simulink model "PerfectModel"  (R2018b)
settings: Solver=VariableStepAuto  StartTime=0.0  StopTime=25  RelTol=1e-3
settings Model: Creator=olavoie  LastModifiedBy=olavoie

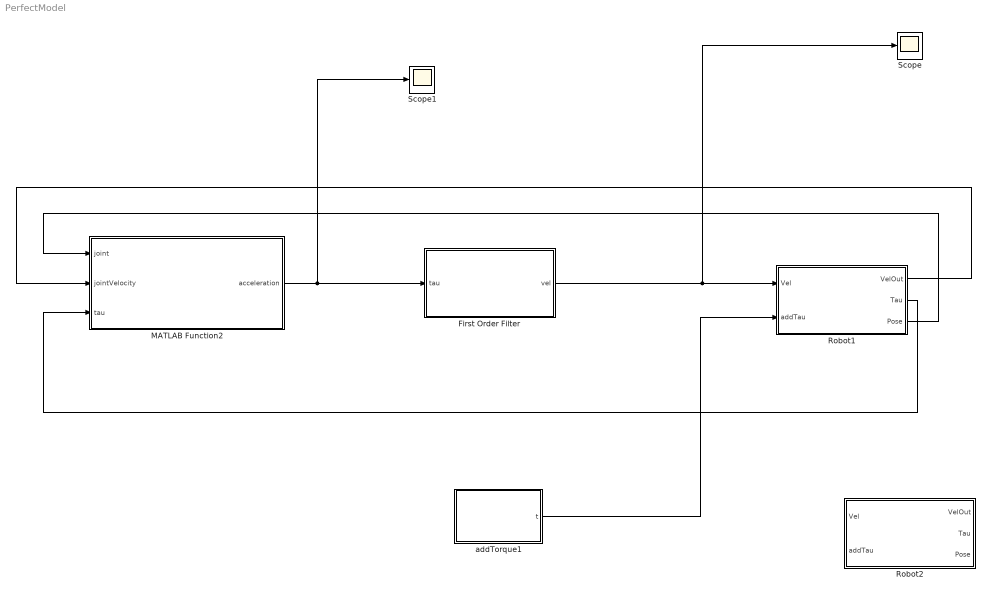
== system PerfectModel ==
  First Order Filter : Subsystem  TreatAsAtomicUnit=on
  MATLAB Function2 : MATLAB Function  TreatAsAtomicUnit=on
  Robot1 : Subsystem  TreatAsAtomicUnit=on
  Robot2 : Subsystem  TreatAsAtomicUnit=on
  Scope : Scope
  Scope1 : Scope
  addTorque1 : Subsystem  TreatAsAtomicUnit=on
  wires:
  MATLAB Function2/1(acceleration) -> Scope1/1, First Order Filter/1(tau)
  First Order Filter/1(vel) -> Scope/1, Robot1/1(Vel)
  Robot1/1(VelOut) -> MATLAB Function2/2(jointVelocity)
  Robot1/3(Pose) -> MATLAB Function2/1(joint)
  Robot1/2(Tau) -> MATLAB Function2/3(tau)
  addTorque1/1(t) -> Robot1/2(addTau)

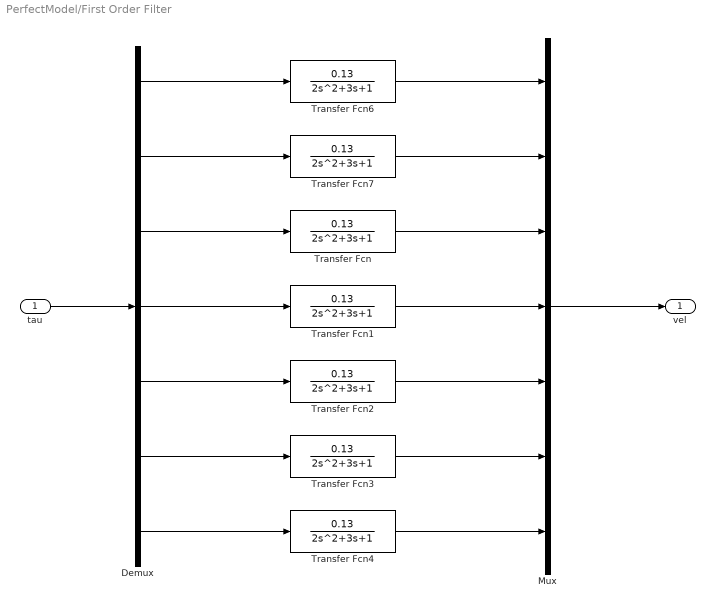
== system PerfectModel/First Order Filter ==
  tau : Inport
  Demux : Demux  Outputs=7
  Mux : Mux  Inputs=7
  Transfer Fcn{,1..4,6..7} (7 alike) : TransferFcn  Numerator=[0.13]  Denominator=[2 3 1]
  vel : Outport
  wires:
  Transfer Fcn2/1 -> Mux/5
  Demux/7 -> Transfer Fcn4/1
  Transfer Fcn1/1 -> Mux/4
  Transfer Fcn4/1 -> Mux/7
  Transfer Fcn/1 -> Mux/3
  Demux/3 -> Transfer Fcn/1
  Demux/5 -> Transfer Fcn2/1
  Transfer Fcn7/1 -> Mux/2
  Transfer Fcn3/1 -> Mux/6
  Mux/1 -> vel/1
  Demux/4 -> Transfer Fcn1/1
  tau/1 -> Demux/1
  Demux/6 -> Transfer Fcn3/1
  Transfer Fcn6/1 -> Mux/1
  Demux/2 -> Transfer Fcn7/1
  Demux/1 -> Transfer Fcn6/1

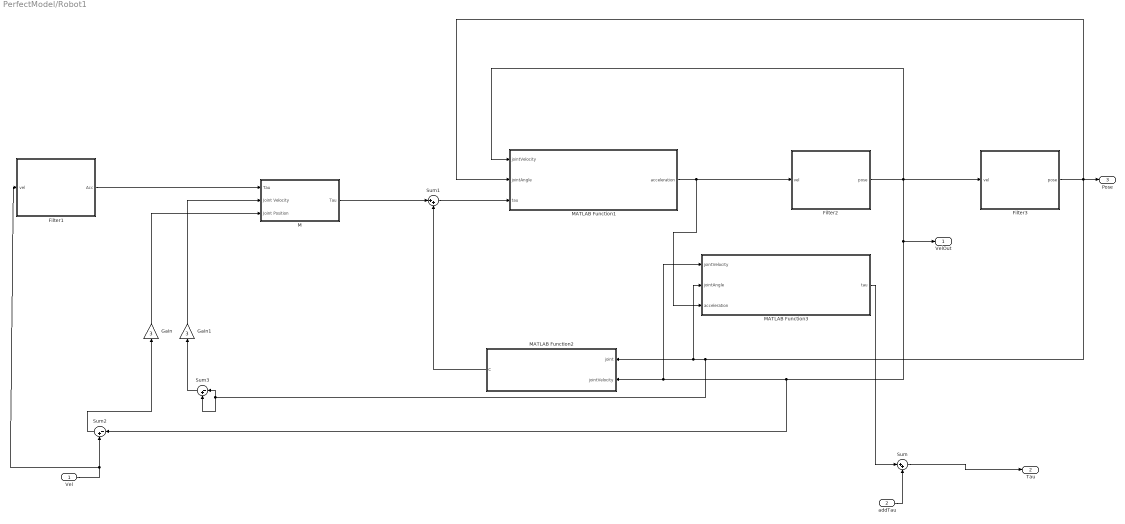
== system PerfectModel/Robot1 ==
  Vel : Inport
  addTau : Inport  Port=2
  Filter1 : Subsystem  TreatAsAtomicUnit=on
  Filter2 : Subsystem  TreatAsAtomicUnit=on
  Filter3 : Subsystem  TreatAsAtomicUnit=on
  Gain : Gain  Gain=3
  Gain1 : Gain  Gain=3
  M : Subsystem  TreatAsAtomicUnit=on
  MATLAB Function1 : MATLAB Function  TreatAsAtomicUnit=on
  MATLAB Function2 : MATLAB Function  TreatAsAtomicUnit=on
  MATLAB Function3 : MATLAB Function  TreatAsAtomicUnit=on
  Sum : Sum  Inputs=|++
  Sum1 : Sum  Inputs=|++
  Sum2 : Sum  Inputs=|-+
  Sum3 : Sum  Inputs=|-+
  VelOut : Outport
  Tau : Outport  Port=2
  Pose : Outport  Port=3
  wires:
  Sum1/1 -> MATLAB Function1/3(tau)
  MATLAB Function1/1(acceleration) -> MATLAB Function3/3(acceleration), Filter2/1(vel)
  Filter2/1(pose) -> VelOut/1, Sum2/1, MATLAB Function3/1(jointVelocity), MATLAB Function2/2(jointVelocity), Filter3/1(vel), MATLAB Function1/1(jointVelocity)
  Filter3/1(pose) -> Sum3/2, Sum3/1, MATLAB Function3/2(jointAngle), MATLAB Function2/1(joint), MATLAB Function1/2(jointAngle), Pose/1
  addTau/1 -> Sum/2
  Sum/1 -> Tau/1
  M/1(Tau) -> Sum1/1
  MATLAB Function2/1(C) -> Sum1/2
  Sum3/1 -> Gain1/1
  Gain1/1 -> M/2(Joint Velocity)
  Sum2/1 -> Gain/1
  Gain/1 -> M/3(Joint Position)
  Vel/1 -> Filter1/1(vel), Sum2/2
  Filter1/1(Acc) -> M/1("Tau ")
  MATLAB Function3/1(tau) -> Sum/1

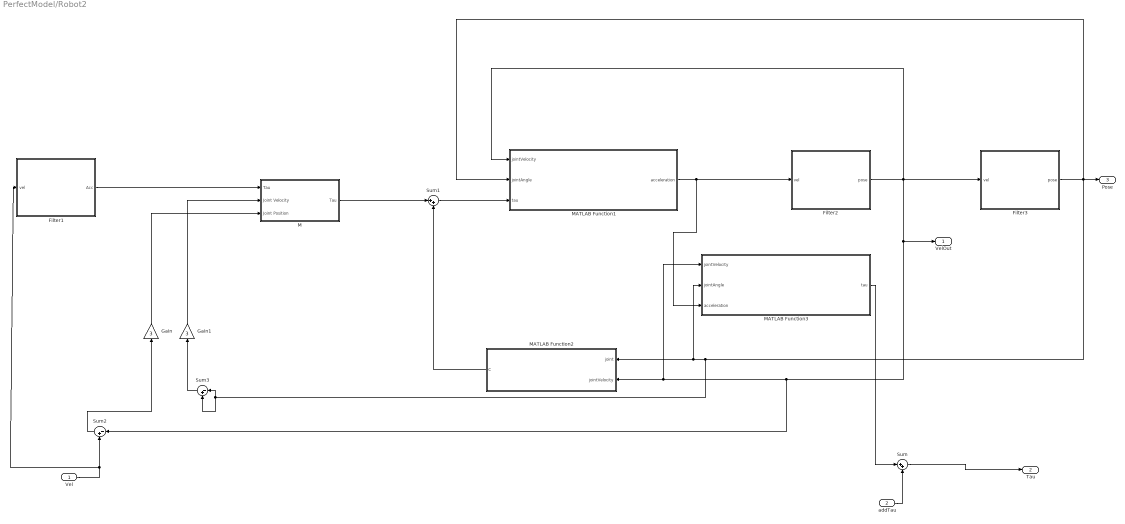
== system PerfectModel/Robot2 ==
  Vel : Inport
  addTau : Inport  Port=2
  Filter1 : Subsystem  TreatAsAtomicUnit=on
  Filter2 : Subsystem  TreatAsAtomicUnit=on
  Filter3 : Subsystem  TreatAsAtomicUnit=on
  Gain : Gain  Gain=3
  Gain1 : Gain  Gain=3
  M : Subsystem  TreatAsAtomicUnit=on
  MATLAB Function1 : MATLAB Function  TreatAsAtomicUnit=on
  MATLAB Function2 : MATLAB Function  TreatAsAtomicUnit=on
  MATLAB Function3 : MATLAB Function  TreatAsAtomicUnit=on
  Sum : Sum  Inputs=|++
  Sum1 : Sum  Inputs=|++
  Sum2 : Sum  Inputs=|-+
  Sum3 : Sum  Inputs=|-+
  VelOut : Outport
  Tau : Outport  Port=2
  Pose : Outport  Port=3
  wires:
  Sum1/1 -> MATLAB Function1/3(tau)
  MATLAB Function1/1(acceleration) -> MATLAB Function3/3(acceleration), Filter2/1(vel)
  Filter2/1(pose) -> VelOut/1, Sum2/1, MATLAB Function3/1(jointVelocity), MATLAB Function2/2(jointVelocity), Filter3/1(vel), MATLAB Function1/1(jointVelocity)
  Filter3/1(pose) -> Sum3/2, Sum3/1, MATLAB Function3/2(jointAngle), MATLAB Function2/1(joint), MATLAB Function1/2(jointAngle), Pose/1
  addTau/1 -> Sum/2
  Sum/1 -> Tau/1
  M/1(Tau) -> Sum1/1
  MATLAB Function2/1(C) -> Sum1/2
  Sum3/1 -> Gain1/1
  Gain1/1 -> M/2(Joint Velocity)
  Sum2/1 -> Gain/1
  Gain/1 -> M/3(Joint Position)
  Vel/1 -> Filter1/1(vel), Sum2/2
  Filter1/1(Acc) -> M/1("Tau ")
  MATLAB Function3/1(tau) -> Sum/1

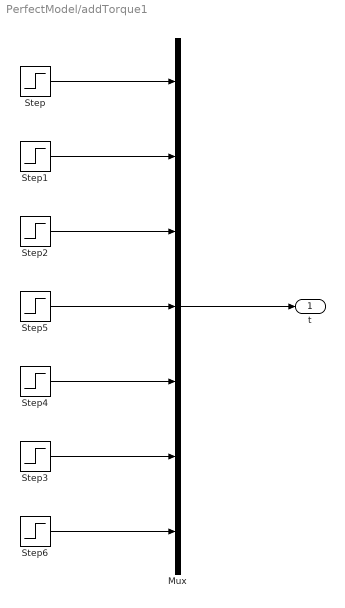
== system PerfectModel/addTorque1 ==
  Mux : Mux  Inputs=7
  Step : Step  After=100  SampleTime=0
  Step1 : Step  Time=0  After=0  SampleTime=0
  Step{2..3,5..6} (4 alike) : Step  After=0  SampleTime=0
  Step4 : Step  Time=0  After=0  SampleTime=0
  t : Outport
  wires:
  Step1/1 -> Mux/2
  Step2/1 -> Mux/3
  Step5/1 -> Mux/4
  Step4/1 -> Mux/5
  Step3/1 -> Mux/6
  Step6/1 -> Mux/7
  Step/1 -> Mux/1
  Mux/1 -> t/1

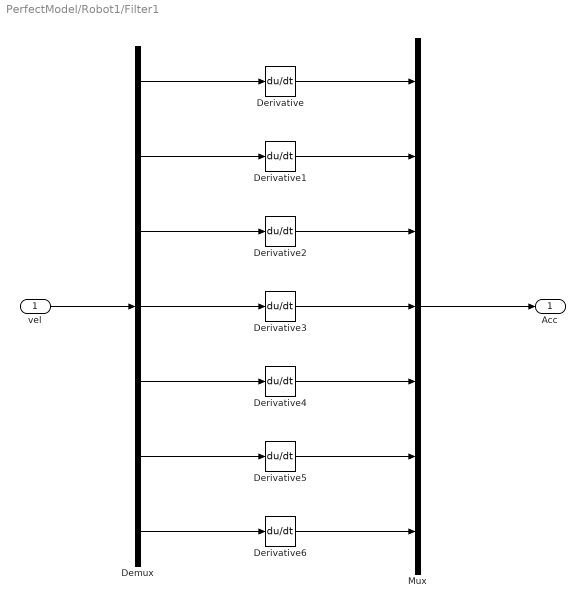
== system PerfectModel/Robot1/Filter1 ==
  vel : Inport
  Demux : Demux  Outputs=7
  Derivative{,1..6} (7 alike) : Derivative
  Mux : Mux  Inputs=7
  Acc : Outport
  wires:
  Mux/1 -> Acc/1
  Demux/1 -> Derivative/1
  Derivative/1 -> Mux/1
  Demux/7 -> Derivative6/1
  Derivative6/1 -> Mux/7
  Demux/6 -> Derivative5/1
  Derivative5/1 -> Mux/6
  Demux/5 -> Derivative4/1
  Derivative4/1 -> Mux/5
  Demux/4 -> Derivative3/1
  Derivative3/1 -> Mux/4
  Demux/3 -> Derivative2/1
  Derivative2/1 -> Mux/3
  Demux/2 -> Derivative1/1
  Derivative1/1 -> Mux/2
  vel/1 -> Demux/1

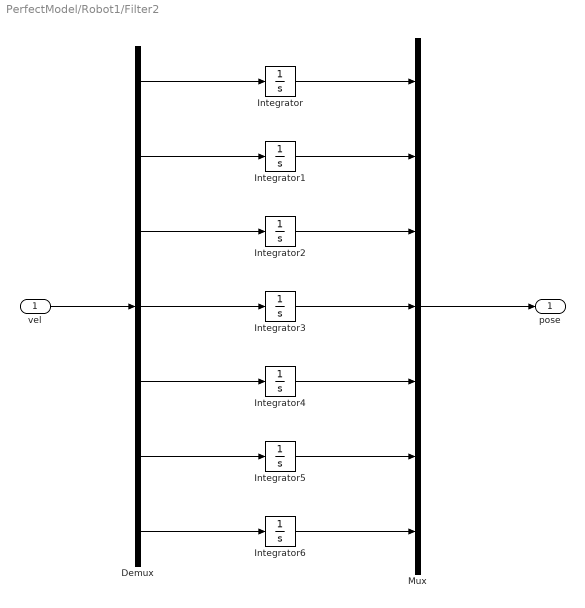
== system PerfectModel/Robot1/Filter2 ==
  vel : Inport
  Demux : Demux  Outputs=7
  Integrator{,1..6} (7 alike) : Integrator
  Mux : Mux  Inputs=7
  pose : Outport
  wires:
  Mux/1 -> pose/1
  Demux/1 -> Integrator/1
  Integrator/1 -> Mux/1
  Demux/7 -> Integrator6/1
  Integrator6/1 -> Mux/7
  Demux/6 -> Integrator5/1
  Integrator5/1 -> Mux/6
  Demux/5 -> Integrator4/1
  Integrator4/1 -> Mux/5
  Demux/4 -> Integrator3/1
  Integrator3/1 -> Mux/4
  Demux/3 -> Integrator2/1
  Integrator2/1 -> Mux/3
  Demux/2 -> Integrator1/1
  Integrator1/1 -> Mux/2
  vel/1 -> Demux/1

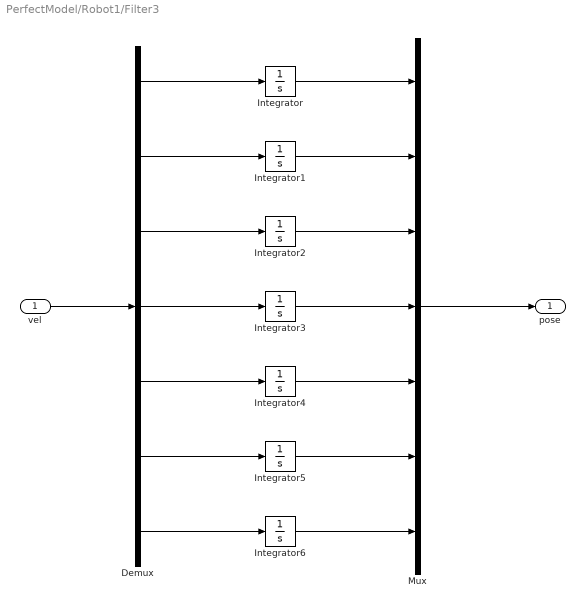
== system PerfectModel/Robot1/Filter3 ==
  vel : Inport
  Demux : Demux  Outputs=7
  Integrator{,1..6} (7 alike) : Integrator
  Mux : Mux  Inputs=7
  pose : Outport
  wires:
  Mux/1 -> pose/1
  Demux/1 -> Integrator/1
  Integrator/1 -> Mux/1
  Demux/7 -> Integrator6/1
  Integrator6/1 -> Mux/7
  Demux/6 -> Integrator5/1
  Integrator5/1 -> Mux/6
  Demux/5 -> Integrator4/1
  Integrator4/1 -> Mux/5
  Demux/4 -> Integrator3/1
  Integrator3/1 -> Mux/4
  Demux/3 -> Integrator2/1
  Integrator2/1 -> Mux/3
  Demux/2 -> Integrator1/1
  Integrator1/1 -> Mux/2
  vel/1 -> Demux/1

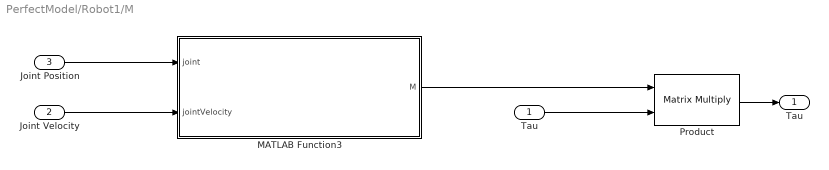
== system PerfectModel/Robot1/M ==
  "Tau " : Inport
  Joint Velocity : Inport  Port=2
  Joint Position : Inport  Port=3
  MATLAB Function3 : MATLAB Function  TreatAsAtomicUnit=on
  Product : Product  Multiplication=Matrix(*)
  Tau : Outport
  wires:
  MATLAB Function3/1(M) -> Product/1
  Product/1 -> Tau/1
  Joint Position/1 -> MATLAB Function3/1(joint)
  Joint Velocity/1 -> MATLAB Function3/2(jointVelocity)
  "Tau "/1 -> Product/2

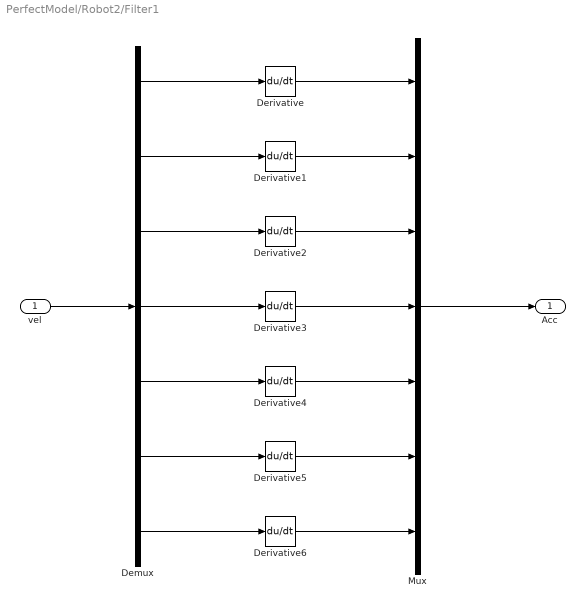
== system PerfectModel/Robot2/Filter1 ==
  vel : Inport
  Demux : Demux  Outputs=7
  Derivative{,1..6} (7 alike) : Derivative
  Mux : Mux  Inputs=7
  Acc : Outport
  wires:
  Mux/1 -> Acc/1
  Demux/1 -> Derivative/1
  Derivative/1 -> Mux/1
  Demux/7 -> Derivative6/1
  Derivative6/1 -> Mux/7
  Demux/6 -> Derivative5/1
  Derivative5/1 -> Mux/6
  Demux/5 -> Derivative4/1
  Derivative4/1 -> Mux/5
  Demux/4 -> Derivative3/1
  Derivative3/1 -> Mux/4
  Demux/3 -> Derivative2/1
  Derivative2/1 -> Mux/3
  Demux/2 -> Derivative1/1
  Derivative1/1 -> Mux/2
  vel/1 -> Demux/1

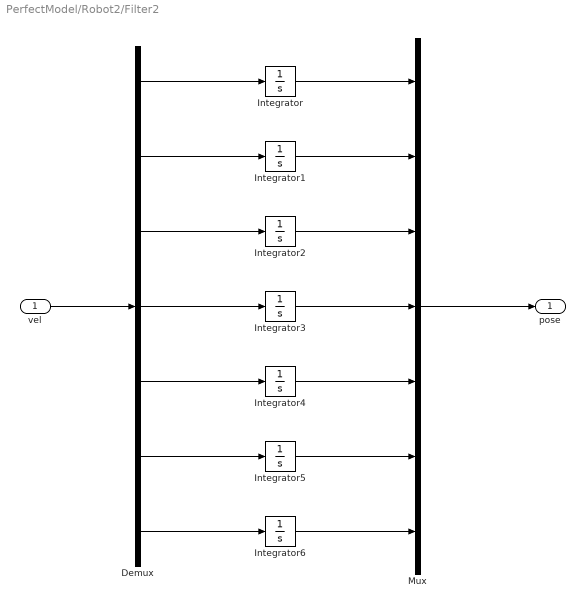
== system PerfectModel/Robot2/Filter2 ==
  vel : Inport
  Demux : Demux  Outputs=7
  Integrator{,1..6} (7 alike) : Integrator
  Mux : Mux  Inputs=7
  pose : Outport
  wires:
  Mux/1 -> pose/1
  Demux/1 -> Integrator/1
  Integrator/1 -> Mux/1
  Demux/7 -> Integrator6/1
  Integrator6/1 -> Mux/7
  Demux/6 -> Integrator5/1
  Integrator5/1 -> Mux/6
  Demux/5 -> Integrator4/1
  Integrator4/1 -> Mux/5
  Demux/4 -> Integrator3/1
  Integrator3/1 -> Mux/4
  Demux/3 -> Integrator2/1
  Integrator2/1 -> Mux/3
  Demux/2 -> Integrator1/1
  Integrator1/1 -> Mux/2
  vel/1 -> Demux/1

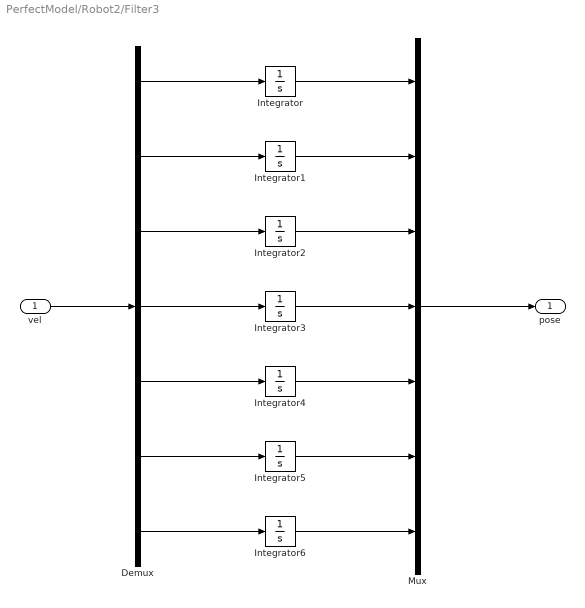
== system PerfectModel/Robot2/Filter3 ==
  vel : Inport
  Demux : Demux  Outputs=7
  Integrator{,1..6} (7 alike) : Integrator
  Mux : Mux  Inputs=7
  pose : Outport
  wires:
  Mux/1 -> pose/1
  Demux/1 -> Integrator/1
  Integrator/1 -> Mux/1
  Demux/7 -> Integrator6/1
  Integrator6/1 -> Mux/7
  Demux/6 -> Integrator5/1
  Integrator5/1 -> Mux/6
  Demux/5 -> Integrator4/1
  Integrator4/1 -> Mux/5
  Demux/4 -> Integrator3/1
  Integrator3/1 -> Mux/4
  Demux/3 -> Integrator2/1
  Integrator2/1 -> Mux/3
  Demux/2 -> Integrator1/1
  Integrator1/1 -> Mux/2
  vel/1 -> Demux/1

== system PerfectModel/Robot2/M ==
  "Tau " : Inport
  Joint Velocity : Inport  Port=2
  Joint Position : Inport  Port=3
  MATLAB Function3 : MATLAB Function  TreatAsAtomicUnit=on
  Product : Product  Multiplication=Matrix(*)
  Tau : Outport
  wires:
  MATLAB Function3/1(M) -> Product/1
  Product/1 -> Tau/1
  Joint Position/1 -> MATLAB Function3/1(joint)
  Joint Velocity/1 -> MATLAB Function3/2(jointVelocity)
  "Tau "/1 -> Product/2

== matlab function PerfectModel/Robot1/M/MATLAB Function3 ==
  data: joint input; M output; jointVelocity input
function M = MassMatrix(joint, jointVelocity)
     M = zeros(7,7);
     
     C = InverseDynamic(jointVelocity, joint, [0; 0; 0; 0; 0; 0; 0]);
     
     for n = 1:7
        a = [0; 0; 0; 0; 0; 0; 0];
        a(n) = 1;
        M(:, n) = InverseDynamic(jointVelocity,joint ,a) - C;
     end 
end

== matlab function PerfectModel/Robot1/MATLAB Function1 ==
  data: jointVelocity input; acceleration output; jointAngle input; tau input
function acceleration = ForwardDynamicSolver(jointVelocity, jointAngle, tau)
    acceleration = ForwardDynamicSolver(jointVelocity, jointAngle, tau);
end

== matlab function PerfectModel/MATLAB Function2 ==
  data: joint input; acceleration output; jointVelocity input; tau input
function acceleration = ForwardDynamicSolver(joint, jointVelocity, tau)
     acceleration = ForwardDynamicSolver(jointVelocity, joint, tau);
end

== matlab function PerfectModel/Robot1/MATLAB Function3 ==
  data: jointVelocity input; tau output; jointAngle input; acceleration input
function tau = ForwardDynamicSolver(jointVelocity, jointAngle, acceleration)
    tau = InverseDynamic(jointVelocity, jointAngle, acceleration);
end

== matlab function PerfectModel/Robot2/M/MATLAB Function3 ==
  data: joint input; M output; jointVelocity input
function M = MassMatrix(joint, jointVelocity)
     M = zeros(7,7);
     
     C = InverseDynamic(jointVelocity, joint, [0; 0; 0; 0; 0; 0; 0]);
     
     for n = 1:7
        a = [0; 0; 0; 0; 0; 0; 0];
        a(n) = 1;
        M(:, n) = InverseDynamic(jointVelocity,joint ,a) - C;
     end 
end

== matlab function PerfectModel/Robot1/MATLAB Function2 ==
  data: joint input; C output; jointVelocity input
function C = SystemCompensation(joint, jointVelocity)
     
     C = InverseDynamic(jointVelocity, joint, [0; 0; 0; 0; 0; 0; 0]);
end

== matlab function PerfectModel/Robot2/MATLAB Function1 ==
  data: jointVelocity input; acceleration output; jointAngle input; tau input
function acceleration = ForwardDynamicSolver(jointVelocity, jointAngle, tau)
    acceleration = ForwardDynamicSolver(jointVelocity, jointAngle, tau);
end

== matlab function PerfectModel/Robot2/MATLAB Function2 ==
  data: joint input; C output; jointVelocity input
function C = SystemCompensation(joint, jointVelocity)
     
     C = InverseDynamic(jointVelocity, joint, [0; 0; 0; 0; 0; 0; 0]);
end

== matlab function PerfectModel/Robot2/MATLAB Function3 ==
  data: jointVelocity input; tau output; jointAngle input; acceleration input
function tau = ForwardDynamicSolver(jointVelocity, jointAngle, acceleration)
    tau = InverseDynamic(jointVelocity, jointAngle, acceleration);
end
